simulink model "waypoint_generation_ptCloud_200630_waypoint_filtering_2"  (R2020a)
settings: Solver=ode4  StartTime=0.0  StopTime=200  FixedStep=0.01  RelTol=1e-3  EnableMultiTasking=on
InitFcn:
  | detector = load('ptOPDetector.mat');
  | OPdetector = detector.OPdetector;
undefined symbols (not defined in the file): g, Kd_p, Kd_q, Kd_r, Kd_vx, Kd_vy, Kd_vz, Kff_r, Kff_vx, Kff_vy, Kff_vz, Ki_p, Ki_q, Ki_r, Ki_vx, Ki_vy, Ki_vz, Kp_p, Kp_phi, Kp_psi, Kp_q, Kp_r, Kp_theta, Kp_vx, Kp_vy, Kp_vz, M, pointCloud_center, sigma_motor, w_h
libraries: visiontextngfix x4, sharedtransform x1, shared6dof x1, simulink_extras x1
(part 2 of 2)

== matlab function waypoint_generation_ptCloud_200630_waypoint_filtering_2/3D A* Algorithm/MATLAB Function11 ==
  settings: updateMethod=DISCRETE
  data: pos_grid input; waypoint_given input; point_cmd output; waypoint_gen input; auto_flag output; waypoint_set output
function [point_cmd,auto_flag,waypoint_set] = gen_waypoint(pos_grid,waypoint_given,waypoint_gen)

persistent flag autonomous_mode_flag waypoint_old waypoint_pre

if isempty(flag)
    flag = 1;
end
if isempty(autonomous_mode_flag)
    autonomous_mode_flag = 0;
end
if isempty(waypoint_old)
    waypoint_old = nan(20,3);
end
if isempty(waypoint_pre)
    waypoint_pre = nan(20,3);
    for aaa = 1:numel(waypoint_given)/3
        waypoint_pre(aaa,:)=waypoint_given(aaa,:);
    end
end
pos_grid = int32(pos_grid);
waypoint_pre_x = waypoint_pre(:,1);
waypoint_pre_y = waypoint_pre(:,2);
waypoint_pre_z = waypoint_pre(:,3);

point_cmd_temp = int32([waypoint_pre_x(flag) waypoint_pre_y(flag) waypoint_pre_z(flag)]);
waypoint_auto_set = nan(40,3);
waypoint_distance = nan(40,1);

if autonomous_mode_flag==0
    if abs(point_cmd_temp(1)-pos_grid(1)) <= 0 && abs(point_cmd_temp(2)-pos_grid(2)) <= 0 && abs(point_cmd_temp(3)-pos_grid(3)) <= 0
        flag = flag + 1;
        
        if flag == numel(rmmissing(waypoint_pre))/3 + 1
            flag = numel(rmmissing(waypoint_pre))/3;
            autonomous_mode_flag = 1;
        end
    end
    
    % waypoint_gen_filtered = rmmissing(waypoint_gen);
    % if ~isempty(waypoint_gen_filtered)
    %     if flag == numel(waypoint_pre)/3
    %         waypoint_x = waypoint_gen_filtered(1,1);
    %         waypoint_y = waypoint_gen_filtered(1,2);
    %         waypoint_z = waypoint_gen_filtered(1,3);
    %     end
    % end
elseif autonomous_mode_flag==1
    waypoint_auto_old = rmmissing(waypoint_old);
    waypoint_auto_new = rmmissing(waypoint_gen);
    if isempty(waypoint_auto_old)
        waypoint_auto_old = waypoint_auto_new;
    end
    
    if ~isempty(waypoint_auto_old) && ~isempty(waypoint_auto_new)
        for mmm = numel(waypoint_auto_new)/3:-1:1
            changed_flag=0;
            for nnn = 1:numel(waypoint_auto_old)/3
                if ((waypoint_auto_new(mmm,1)-waypoint_auto_old(nnn,1))^2+(waypoint_auto_new(mmm,2)-waypoint_auto_old(nnn,2))^2+(waypoint_auto_new(mmm,3)-waypoint_auto_old(nnn,3))^2)<900
                    waypoint_auto_old(nnn,:)=waypoint_auto_new(mmm,:);
                    changed_flag=1;
                end
            end
            if changed_flag == 1
                waypoint_auto_new(mmm,:)=nan(1,3);
            end
        end
%         waypoint_auto_set_temp = cat(1,unique(waypoint_auto_old,'stable','rows'),waypoint_auto_new);

%             waypoint_auto_set_temp = rmmissing(cat(1,waypoint_auto_new,unique(waypoint_auto_old,'stable','rows')));
            waypoint_auto_set_temp = rmmissing(cat(1,unique(waypoint_auto_old,'stable','rows'),waypoint_auto_new));

        
        for aaa = 1:numel(waypoint_auto_set_temp)/3
            waypoint_auto_set(aaa,:)=waypoint_auto_set_temp(aaa,:);
            waypoint_distance(aaa) = (((waypoint_auto_set(aaa,1)-pos_grid(1))^2+(waypoint_auto_set(aaa,2)-pos_grid(2))^2+(waypoint_auto_set(aaa,3)-pos_grid(3))^2));
        end
        [~,waypoint_index]=sort(waypoint_distance);
        
        for aaa = 1:length(waypoint_index)
            waypoint_auto_set(aaa,:)=waypoint_auto_set(waypoint_index(aaa),:);
        end
%         waypoint_auto_set(1:aaa,:)=waypoint_auto_set_temp(waypoint_index,:);
        
        point_cmd_temp = int32([waypoint_auto_set(1,1), waypoint_auto_set(1,2), waypoint_auto_set(1,3)]);
        
        if abs(point_cmd_temp(1)-pos_grid(1)) <= 0 && abs(point_cmd_temp(2)-pos_grid(2)) <= 0 && abs(point_cmd_temp(3)-pos_grid(3)) <= 0
            waypoint_auto_set = [waypoint_auto_set(2:end,:); nan(1,3)];            
        end
        
        waypoint_old = waypoint_auto_set(1:20,:);
        
        
    else
        if ~isnan(waypoint_old(1,1)) && ~isnan(waypoint_old(1,2)) && ~isnan(waypoint_old(1,3))
            point_cmd_temp = int32([waypoint_old(1,1), waypoint_old(1,2), waypoint_old(1,3)]);
%             waypoint_pre = waypoint_old;
%             autonomous_mode_flag = 0;
%             flag = 1;

            if abs(point_cmd_temp(1)-pos_grid(1)) <= 0 && abs(point_cmd_temp(2)-pos_grid(2)) <= 0 && abs(point_cmd_temp(3)-pos_grid(3)) <= 0
                waypoint_old = [waypoint_old(2:end,:); nan(1,3)];            
            end


        else
            point_cmd_temp = int32([pos_grid(1), pos_grid(2), pos_grid(3)]);
        end
    end
end


% point_cmd = int32([waypoint_pre_x(flag) waypoint_pre_y(flag) waypoint_pre_z(flag)]);
point_cmd = point_cmd_temp;


auto_flag = autonomous_mode_flag;
waypoint_set = waypoint_auto_set;


end

== matlab function waypoint_generation_ptCloud_200630_waypoint_filtering_2/3D A* Algorithm/MATLAB Function12 ==
  data: odom_input input; pos_grid output; pos_init input
function pos_grid = odom_grid(odom_input,pos_init)

odom = zeros(1,3);
odom(1,1) = odom_input(1);
odom(1,2) = odom_input(2);
odom(1,3) = odom_input(3);

start_point = [pos_init(1) pos_init(2) pos_init(3)];

% pos_x = int16(odom(1)/0.2+0.5);
% pos_y = int16(odom(2)/0.2+0.5);
% pos_z = int16(odom(3)/0.2+0.5);
pos_x = int16(odom(1)/0.2);
pos_y = int16(odom(2)/0.2);
pos_z = int16(odom(3)/0.2);

pos_grid = [pos_x+start_point(1) pos_y+start_point(2) pos_z+start_point(3)];

end

== matlab function waypoint_generation_ptCloud_200630_waypoint_filtering_2/3D A* Algorithm/MATLAB Function6 ==
  data: pos_init input; openpoint_front input; waypoint_gen output; openpoint_back input; openpoint_left input; openpoint_right input
function waypoint_gen = fcn(pos_init,openpoint_front,openpoint_back,openpoint_left,openpoint_right)
grid_size = 0.2;

openpoint_front_grid = int16(openpoint_front/grid_size);
openpoint_back_grid = int16(openpoint_back/grid_size);
openpoint_left_grid = int16(openpoint_left/grid_size);
openpoint_right_grid = int16(openpoint_right/grid_size);

waypoint_gen_front = nan(5,3);
waypoint_gen_back = nan(5,3);
waypoint_gen_left = nan(5,3);
waypoint_gen_right = nan(5,3);

for aaa = 1:5
    if ~isnan(openpoint_front(aaa,1))
        waypoint_gen_front(aaa,:) = [openpoint_front_grid(aaa,1)+int16(pos_init(1)), openpoint_front_grid(aaa,2)+int16(pos_init(2)), openpoint_front_grid(aaa,3)+int16(pos_init(3))];
    end
    if ~isnan(openpoint_back(aaa,1))
        waypoint_gen_back(aaa,:) = [openpoint_back_grid(aaa,1)+int16(pos_init(1)), openpoint_back_grid(aaa,2)+int16(pos_init(2)), openpoint_back_grid(aaa,3)+int16(pos_init(3))];
    end
    if ~isnan(openpoint_left(aaa,1))
        waypoint_gen_left(aaa,:) = [openpoint_left_grid(aaa,1)+int16(pos_init(1)), openpoint_left_grid(aaa,2)+int16(pos_init(2)), openpoint_left_grid(aaa,3)+int16(pos_init(3))];
    end
    if ~isnan(openpoint_right(aaa,1))
        waypoint_gen_right(aaa,:) = [openpoint_right_grid(aaa,1)+int16(pos_init(1)), openpoint_right_grid(aaa,2)+int16(pos_init(2)), openpoint_right_grid(aaa,3)+int16(pos_init(3))];
    end
end

waypoint_gen = [waypoint_gen_front;waypoint_gen_back;waypoint_gen_left;waypoint_gen_right];

== matlab function waypoint_generation_ptCloud_200630_waypoint_filtering_2/3D A* Algorithm/MATLAB Function9 ==
  data: bboxes_raw input; bboxes output; bboxes_size input
function bboxes = fcn(bboxes_raw,bboxes_size)
bboxes = zeros(5,4);
% bboxes_nonzeros = nonzeros(bboxes_raw);
% num_bboxes = min(numel(bboxes_nonzeros)/4,5);
num_bboxes = bboxes_size(1);

if num_bboxes>0
    for aaa = 1:num_bboxes
        bboxes(aaa,:) = [bboxes_raw(aaa+0*num_bboxes),bboxes_raw(aaa+1*num_bboxes),bboxes_raw(aaa+2*num_bboxes),bboxes_raw(aaa+3*num_bboxes)];
%         bboxes(aaa,:) = [bboxes_nonzeros(aaa+0*num_bboxes),bboxes_nonzeros(aaa+1*num_bboxes),bboxes_nonzeros(aaa+2*num_bboxes),bboxes_nonzeros(aaa+3*num_bboxes)];
    end
end
% bboxes(1:num_bboxes,:) = reshape(bboxes_nonzeros,num_bboxes,4);

== matlab function waypoint_generation_ptCloud_200630_waypoint_filtering_2/3D A* Algorithm/MATLAB Function10 ==
  data: bboxes_raw input; bboxes output; bboxes_size input
function bboxes = fcn(bboxes_raw,bboxes_size)
bboxes = zeros(5,4);
% bboxes_nonzeros = nonzeros(bboxes_raw);
% num_bboxes = min(numel(bboxes_nonzeros)/4,5);
num_bboxes = bboxes_size(1);

if num_bboxes>0
    for aaa = 1:num_bboxes
        bboxes(aaa,:) = [bboxes_raw(aaa+0*num_bboxes),bboxes_raw(aaa+1*num_bboxes),bboxes_raw(aaa+2*num_bboxes),bboxes_raw(aaa+3*num_bboxes)];
%         bboxes(aaa,:) = [bboxes_nonzeros(aaa+0*num_bboxes),bboxes_nonzeros(aaa+1*num_bboxes),bboxes_nonzeros(aaa+2*num_bboxes),bboxes_nonzeros(aaa+3*num_bboxes)];
    end
end
% bboxes(1:num_bboxes,:) = reshape(bboxes_nonzeros,num_bboxes,4);

== matlab function waypoint_generation_ptCloud_200630_waypoint_filtering_2/3D A* Algorithm/MATLAB Function13 ==
  data: bboxes_raw input; bboxes output; bboxes_size input
function bboxes = fcn(bboxes_raw,bboxes_size)
bboxes = zeros(5,4);
% bboxes_nonzeros = nonzeros(bboxes_raw);
% num_bboxes = min(numel(bboxes_nonzeros)/4,5);
num_bboxes = bboxes_size(1);

if num_bboxes>0
    for aaa = 1:num_bboxes
        bboxes(aaa,:) = [bboxes_raw(aaa+0*num_bboxes),bboxes_raw(aaa+1*num_bboxes),bboxes_raw(aaa+2*num_bboxes),bboxes_raw(aaa+3*num_bboxes)];
%         bboxes(aaa,:) = [bboxes_nonzeros(aaa+0*num_bboxes),bboxes_nonzeros(aaa+1*num_bboxes),bboxes_nonzeros(aaa+2*num_bboxes),bboxes_nonzeros(aaa+3*num_bboxes)];
    end
end
% bboxes(1:num_bboxes,:) = reshape(bboxes_nonzeros,num_bboxes,4);

== matlab function waypoint_generation_ptCloud_200630_waypoint_filtering_2/Generation_Angle_error/Attitude Generation (phi,theta,psi) ==
  data: DCM input; acc_cmd input; angle_error output; R_rp_x output
function [angle_error,R_rp_x]  = fcn(DCM,acc_cmd)
%#codegen

R_z           = DCM(3,:)'; 

% for i = 1:length(R_z)
%     if abs(R_z(i)) < 0.001
%         R_z(i) = 0;
%     end
% end

acc_unit      = R_z     / norm(R_z);
acc_cmd_unit  = acc_cmd / norm(acc_cmd);

angle_error = DCM * cross(acc_unit,acc_cmd_unit); %% e_R , consider phi, theta


% Calculate R_rp_x
angle = atan(norm(cross(acc_unit,acc_cmd_unit))/norm(dot(acc_unit,acc_cmd_unit))); % only phi,theta

e_R = angle_error;
R= DCM';

% e_R_cp matrix cross product
e_R_cp = zeros(3,3);
e_R_cp(1,2) = -e_R(3);
e_R_cp(1,3) =  e_R(2);
e_R_cp(2,1) =  e_R(3);
e_R_cp(2,3) = -e_R(1);
e_R_cp(3,1) = -e_R(2);
e_R_cp(3,2) =  e_R(1);

% Result
R_rp = R*(eye(3,3) + e_R_cp*sin(angle) + e_R_cp*e_R_cp*(1-cos(angle)));
R_rp_x = R_rp(:,1);
% acc_cmd_result = R_rp(:,3);

== matlab function waypoint_generation_ptCloud_200630_waypoint_filtering_2/3D A* Algorithm/MATLAB Function14 ==
  data: bboxes_raw input; bboxes output; bboxes_size input
function bboxes = fcn(bboxes_raw,bboxes_size)
bboxes = zeros(5,4);
% bboxes_nonzeros = nonzeros(bboxes_raw);
% num_bboxes = min(numel(bboxes_nonzeros)/4,5);
num_bboxes = bboxes_size(1);

if num_bboxes>0
    for aaa = 1:num_bboxes
        bboxes(aaa,:) = [bboxes_raw(aaa+0*num_bboxes),bboxes_raw(aaa+1*num_bboxes),bboxes_raw(aaa+2*num_bboxes),bboxes_raw(aaa+3*num_bboxes)];
%         bboxes(aaa,:) = [bboxes_nonzeros(aaa+0*num_bboxes),bboxes_nonzeros(aaa+1*num_bboxes),bboxes_nonzeros(aaa+2*num_bboxes),bboxes_nonzeros(aaa+3*num_bboxes)];
    end
end
% bboxes(1:num_bboxes,:) = reshape(bboxes_nonzeros,num_bboxes,4);

== matlab function waypoint_generation_ptCloud_200630_waypoint_filtering_2/3D A* Algorithm/MATLAB Function7 ==
  settings: updateMethod=DISCRETE
  data: pos_current input; optimal_path_x output size=[128 1]; point_cmd input; Obstacle input; pos_init input; optimal_path_y output size=[128 1]; optimal_path_z output size=[128 1]
function [optimal_path_x,optimal_path_y,optimal_path_z] = Astar_algorithm_function(pos_current,point_cmd,Obstacle,pos_init)

persistent optimal sample

if isempty(optimal)
    optimal = nan(128,3);
    sample = 99;
%     sample = 19;
end


sample = sample + 1;

if sample == 100
% if sample == 20
    sample = 1;
    
    mapsize = [150 100 30];
    
    Height = mapsize(1);        % x
    Width = mapsize(2);         % y
    Alt = mapsize(3);            % z
    
    Start = pos_current;
    Goal = point_cmd;
    look = 2;
    H_weight = 1.2;
    
    G_cost = zeros(2*look+1,2*look+1,2*look+1);
    for i = 1:2*look+1
        for j = 1:2*look+1
            for k = 1:2*look+1
                temp = [look+1 look+1 look+1]-[i j k];
                G_cost(i,j,k) = (min(sqrt(sum(abs(temp).^2,2))));
            end
        end
    end
    
    G_top2 = G_cost(:,:,1);
    G_top1 = G_cost(:,:,2);
    G_mid = G_cost(:,:,3);
    G_bottom1 = G_cost(:,:,4);
    G_bottom2 = G_cost(:,:,5);
    
    
    GScore = inf(Height,Width,Alt);
    GScore_temp = zeros(2*look+1,2*look+1,2*look+1);
    HScore = zeros(Height,Width,Alt);
    FScore = inf(Height,Width,Alt);
    ClosedMAT = zeros(Height,Width,Alt);
    CX = int32(Start(1));
    CY = int32(Start(2));
    CZ = int32(Start(3));
    ParentX = inf(Height,Width,Alt);
    ParentY = inf(Height,Width,Alt);
    ParentZ = inf(Height,Width,Alt);
    ParentX(CX,CY,CZ) = CX;
    ParentY(CX,CY,CZ) = CY;
    ParentZ(CX,CY,CZ) = CZ;
    
    %%%%%%%%%%%%%%%% Define Heuristic %%%%%%%%%%%%%%%%%%%%%%%
    for k=1:Alt
        for j=1:Width
            for i=1:Height
                
                temp = (int32(Goal) - int32([i j k])) ;
                Distance=(min(sqrt(sum(abs(temp).^2,2))));
                HScore(i,j,k)=Distance*H_weight;               % (1+sqrt(2))/sqrt(3)
                
            end
        end
    end
    
    FScore(Start(1),Start(2),Start(3)) = HScore(Start(1),Start(2),Start(3));
    GScore(Start(1),Start(2),Start(3)) = 0;
    ClosedMAT(Obstacle==1)=1;
    REACHGOAL = 0;
    
    while 1
        
        MinFScore = min(min(min(FScore)));         % Find Minimun FScore
        if isinf(MinFScore)
            disp('Fail');
            break
        end
        
        
        [minF_x,minF_y] = find(FScore==MinFScore);
        HScore_temp = inf(1,10);
        
        minHScore = 1;
        for i = 1:length(minF_x)
            Current_pose_temp = [minF_x(i) rem(minF_y(i),Width) fix(minF_y(i)/Width)+1];     % H가 가장 적은걸로 먼저 선택
            CX_temp=Current_pose_temp(1);
            CY_temp=Current_pose_temp(2);
            CZ_temp=Current_pose_temp(3);
            HScore_temp(i) = HScore(CX_temp,CY_temp,CZ_temp);
            minHScore = find(HScore_temp == min(HScore_temp));
        end
        
        
        Current_pose = int32([minF_x(minHScore(1)) rem(minF_y(minHScore(1)),Width) fix(minF_y(minHScore(1))/Width)+1]);     % H가 가장 적은걸로 먼저 선택
        CX=Current_pose(1);
        CY=Current_pose(2);
        CZ=Current_pose(3);
        
        
        
        GScore_temp(:,:,1) = GScore(CX,CY,CZ) + G_top2;
        GScore_temp(:,:,2) = GScore(CX,CY,CZ) + G_top1;
        GScore_temp(:,:,3) = GScore(CX,CY,CZ) + G_mid;
        GScore_temp(:,:,4) = GScore(CX,CY,CZ) + G_bottom1;
        GScore_temp(:,:,5) = GScore(CX,CY,CZ) + G_bottom2;
        
        
        
        
        %%%%%%%%%%%%% GScore update %%%%%%%%%%%%%
        
        GScore(CX-look:CX+look,CY-look:CY+look,CZ+2) = min(GScore_temp(:,:,1),GScore(CX-look:CX+look,CY-look:CY+look,CZ+2)) ;
        GScore(CX-look:CX+look,CY-look:CY+look,CZ+1) = min(GScore_temp(:,:,2),GScore(CX-look:CX+look,CY-look:CY+look,CZ+1));
        GScore(CX-look:CX+look,CY-look:CY+look,CZ) = min(GScore_temp(:,:,3), GScore(CX-look:CX+look,CY-look:CY+look,CZ));
        GScore(CX-look:CX+look,CY-look:CY+look,CZ-1) = min(GScore_temp(:,:,4),GScore(CX-look:CX+look,CY-look:CY+look,CZ-1));
        GScore(CX-look:CX+look,CY-look:CY+look,CZ-2) = min(GScore_temp(:,:,5),GScore(CX-look:CX+look,CY-look:CY+look,CZ-2));
        
        
        FScore = GScore + HScore;
        %     ClosedMAT(CX,CY,CZ) = 1;
        ClosedMAT(CX-(look-1):CX+(look-1),CY-(look-1):CY+(look-1),CZ-(look-1):CZ+(look-1)) = 1;
        FScore(ClosedMAT==1) = inf;
        %     Check_FScore = FScore(CX-look:CX+look,CY-look:CY+look,CZ-look:CZ+look);
        
        
        
        [G_row1,G_col1] = find( GScore(CX-look:CX+look,CY-look:CY+look,CZ+2) == GScore_temp(:,:,1) );
        [G_row2,G_col2] = find( GScore(CX-look:CX+look,CY-look:CY+look,CZ+1) == GScore_temp(:,:,2) );
        [G_row3,G_col3] = find( GScore(CX-look:CX+look,CY-look:CY+look,CZ) == GScore_temp(:,:,3) );
        [G_row4,G_col4] = find( GScore(CX-look:CX+look,CY-look:CY+look,CZ-1) == GScore_temp(:,:,4) );
        [G_row5,G_col5] = find( GScore(CX-look:CX+look,CY-look:CY+look,CZ-2) == GScore_temp(:,:,5) );
        
        
        G_row1 = int32(G_row1);
        G_row2 = int32(G_row2);
        G_row3 = int32(G_row3);
        G_row4 = int32(G_row4);
        G_row5 = int32(G_row5);
        
        G_col1 = int32(G_col1);
        G_col2 = int32(G_col2);
        G_col3 = int32(G_col3);
        G_col4 = int32(G_col4);
        G_col5 = int32(G_col5);
        
        G_row1 = G_row1+CX-(look+1);
        G_row2 = G_row2+CX-(look+1);
        G_row3 = G_row3+CX-(look+1);
        G_row4 = G_row4+CX-(look+1);
        G_row5 = G_row5+CX-(look+1);
        
        G_col1 = G_col1+CY-(look+1);
        G_col2 = G_col2+CY-(look+1);
        G_col3 = G_col3+CY-(look+1);
        G_col4 = G_col4+CY-(look+1);
        G_col5 = G_col5+CY-(look+1);
        
        
        for i = 1:length(G_row1)
            ParentX(G_row1(i),G_col1(i),CZ+2) = CX;
            ParentY(G_row1(i),G_col1(i),CZ+2) = CY;
            ParentZ(G_row1(i),G_col1(i),CZ+2) = CZ;
        end
        
        for i = 1:length(G_row2)
            ParentX(G_row2(i),G_col2(i),CZ+1) = CX;
            ParentY(G_row2(i),G_col2(i),CZ+1) = CY;
            ParentZ(G_row2(i),G_col2(i),CZ+1) = CZ;
        end
        
        for i = 1:length(G_row3)
            if G_row3(i)==CX && G_col3(i)==CY
                continue
            end
            ParentX(G_row3(i),G_col3(i),CZ) = CX;
            ParentY(G_row3(i),G_col3(i),CZ) = CY;
            ParentZ(G_row3(i),G_col3(i),CZ) = CZ;
        end
        
        for i = 1:length(G_row4)
            ParentX(G_row4(i),G_col4(i),CZ-1) = CX;
            ParentY(G_row4(i),G_col4(i),CZ-1) = CY;
            ParentZ(G_row4(i),G_col4(i),CZ-1) = CZ;
        end
        
        for i = 1:length(G_row5)
            ParentX(G_row5(i),G_col5(i),CZ-2) = CX;
            ParentY(G_row5(i),G_col5(i),CZ-2) = CY;
            ParentZ(G_row5(i),G_col5(i),CZ-2) = CZ;
        end
        
        
        
        
        if abs(Goal(1)-CX)<=(look-1) && abs(Goal(2)-CY)<=(look-1) && abs(Goal(3)-CZ)<=(look-1)
            REACHGOAL = 1;
            break
        end
        
    end
    
    
    % optimal = nan(128,3);
    if REACHGOAL
        optimal(1,:) = [Goal(1) Goal(2) Goal(3)];
        k=2;
        while 1
            CX_temp = int32(ParentX(CX,CY,CZ));
            CY_temp = int32(ParentY(CX,CY,CZ));
            CZ_temp = int32(ParentZ(CX,CY,CZ));
            
            CX = CX_temp;
            CY = CY_temp;
            CZ = CZ_temp;
            
            optimal(k,:) = [CX CY CZ];
            k = k+1;
            
            if CX==Start(1) && CY==Start(2) && CZ==Start(3)
                break
            end
        end
    end
    
end
start_point = [pos_init(1) pos_init(2) pos_init(3)];

% optimal_path_x = flip(single(((optimal(:,1)-start_point(1))-0.5) * 0.2 + 0.1));      % grid_size = 0.2
% optimal_path_y = flip(single(((optimal(:,2)-start_point(2))-0.5) * 0.2 + 0.1));
% optimal_path_z = flip(single(((optimal(:,3)-start_point(3))-0.5) * 0.2 + 0.1));
optimal_path_x = flip(single( (optimal(:,1)-start_point(1)) * 0.2 ));      % grid_size = 0.2
optimal_path_y = flip(single( (optimal(:,2)-start_point(2)) * 0.2 ));
optimal_path_z = flip(single( (optimal(:,3)-start_point(3)) * 0.2 ));


end

== matlab function waypoint_generation_ptCloud_200630_waypoint_filtering_2/3D A* Algorithm/MATLAB Function8 ==
  data: octomap_center input; Obstacle output; pos_init input
function Obstacle = gen_3d_array(octomap_center,pos_init)

mapsize = [150 100 30];

Obstacle = int8(zeros(mapsize(1),mapsize(2),mapsize(3)));
grid_size = 0.2;
start_point = [pos_init(1) pos_init(2) pos_init(3)];

% align1 = int16(octomap_center/(grid_size)+0.5);
align1 = int16(octomap_center/(grid_size));
align2 = unique(align1,'rows');
align3 = [align2(:,1)+start_point(1) align2(:,2)+start_point(2) align2(:,3)+start_point(3)];

for i = 1:numel(align3)/3
    
    index_temp = align3(i,:);
    
    index_check = index_temp<3;
    if sum(index_check)>=1
        index_temp(index_check) = 3;
    end
    
    if index_temp(1) > mapsize(1)-2
        index_temp(1) = mapsize(1)-2;
    end
    if index_temp(2) > mapsize(2)-2
        index_temp(2) = mapsize(2)-2;
    end
    if index_temp(3) > mapsize(3)-2
        index_temp(3) = mapsize(3)-2;
    end
    

    index_x = index_temp(1)-1:index_temp(1)+1;
    index_y = index_temp(2)-1:index_temp(2)+1;
    index_z = index_temp(3)-1:index_temp(3)+1;

    Obstacle(index_x,index_temp(2)+1,index_temp(3)+1) = 1;
    Obstacle(index_x,index_temp(2)+1,index_temp(3)) = 1;
    Obstacle(index_x,index_temp(2)+1,index_temp(3)-1) = 1;
    Obstacle(index_x,index_temp(2),index_temp(3)+1) = 1;
    Obstacle(index_x,index_temp(2),index_temp(3)) = 1;
    Obstacle(index_x,index_temp(2),index_temp(3)-1) = 1;
    Obstacle(index_x,index_temp(2)-1,index_temp(3)+1) = 1;
    Obstacle(index_x,index_temp(2)-1,index_temp(3)) = 1;
    Obstacle(index_x,index_temp(2)-1,index_temp(3)-1) = 1;
    
%     Obstacle(index_temp(1)+1,index_temp(2)+2,index_z) = 1;
%     Obstacle(index_temp(1)+1,index_temp(2)-2,index_z) = 1;
%     Obstacle(index_temp(1)+1,index_y,index_temp(3)+2) = 1;
%     Obstacle(index_temp(1)+1,index_y,index_temp(3)-2) = 1;
%     Obstacle(index_temp(1),index_temp(2)+2,index_z) = 1;
%     Obstacle(index_temp(1),index_temp(2)-2,index_z) = 1;
%     Obstacle(index_temp(1),index_y,index_temp(3)+2) = 1;
%     Obstacle(index_temp(1),index_y,index_temp(3)-2) = 1;
%     Obstacle(index_temp(1)-1,index_temp(2)+2,index_z) = 1;
%     Obstacle(index_temp(1)-1,index_temp(2)-2,index_z) = 1;
%     Obstacle(index_temp(1)-1,index_y,index_temp(3)+2) = 1;
%     Obstacle(index_temp(1)-1,index_y,index_temp(3)-2) = 1;
    
    
    
    
%     Obstacle(index_temp(1)+2,index_temp(2)+2,index_z) = 1;
%     Obstacle(index_temp(1)+2,index_temp(2)+1,index_z) = 1;
%     Obstacle(index_temp(1)+2,index_temp(2),index_z) = 1;
%     Obstacle(index_temp(1)+2,index_temp(2)-1,index_z) = 1;
%     Obstacle(index_temp(1)+2,index_temp(2)-2,index_z) = 1;
%     
%     Obstacle(index_temp(1)+1,index_temp(2)+2,index_z) = 1;
%     Obstacle(index_temp(1)+1,index_temp(2)+1,index_z) = 1;
%     Obstacle(index_temp(1)+1,index_temp(2),index_z) = 1;
%     Obstacle(index_temp(1)+1,index_temp(2)-1,index_z) = 1;
%     Obstacle(index_temp(1)+1,index_temp(2)-2,index_z) = 1;
%     
%     Obstacle(index_temp(1),index_temp(2)+2,index_z) = 1;
%     Obstacle(index_temp(1),index_temp(2)+1,index_z) = 1;
%     Obstacle(index_temp(1),index_temp(2),index_z) = 1;
%     Obstacle(index_temp(1),index_temp(2)-1,index_z) = 1;
%     Obstacle(index_temp(1),index_temp(2)-2,index_z) = 1;
%     
%     Obstacle(index_temp(1)-1,index_temp(2)+2,index_z) = 1;
%     Obstacle(index_temp(1)-1,index_temp(2)+1,index_z) = 1;
%     Obstacle(index_temp(1)-1,index_temp(2),index_z) = 1;
%     Obstacle(index_temp(1)-1,index_temp(2)-1,index_z) = 1;
%     Obstacle(index_temp(1)-1,index_temp(2)-2,index_z) = 1;
%     
%     Obstacle(index_temp(1)-2,index_temp(2)+2,index_z) = 1;
%     Obstacle(index_temp(1)-2,index_temp(2)+1,index_z) = 1;
%     Obstacle(index_temp(1)-2,index_temp(2),index_z) = 1;
%     Obstacle(index_temp(1)-2,index_temp(2)-1,index_z) = 1;
%     Obstacle(index_temp(1)-2,index_temp(2)-2,index_z) = 1;
    
end

Obstacle(1:3,:,:)=1;
Obstacle(mapsize(1)-2:mapsize(1),:,:) = 1;
Obstacle(:,1:3,:) = 1;
Obstacle(:,mapsize(2)-2:mapsize(2),:) = 1;
Obstacle(:,:,1:3) = 1;
Obstacle(:,:,mapsize(3)-10:mapsize(3)) = 1;

end

== matlab function waypoint_generation_ptCloud_200630_waypoint_filtering_2/Path Guidance/MATLAB Function ==
  data: X_vel_cmd output; Y_vel_cmd output; odom input; Z_vel_cmd output; optimal_path_x input size=[128 1]; optimal_path_y input size=[128 1]; optimal_path_z input size=[128 1]; yaw_cmd output
function [X_vel_cmd,Y_vel_cmd,Z_vel_cmd,yaw_cmd] = fcn(odom,optimal_path_x,optimal_path_y,optimal_path_z)

P_gain = 0.5;

path_length = length(optimal_path_x);
K = inf(path_length,1);
optimal_path_norm = inf(path_length,3);

% optimal_path_x_temp = optimal_path_x.Data';
% optimal_path_y_temp = optimal_path_y.Data';

optimal_path_norm(:,1) = single(optimal_path_x - odom(1));
optimal_path_norm(:,2) = single(optimal_path_y - odom(2));
optimal_path_norm(:,3) = single(optimal_path_z - odom(3));

% optimal_path = [optimal_path_x' optimal_path_y'];
% optimal_path_norm = optimal_path - [odom(1) odom(2)];

for i=1:path_length
    K(i) = norm(optimal_path_norm(i,:));
end

[~,m] = min(K);



% Z_cmd = optimal_path_z(m);
if m >= 128
    m = 127;
end
% Z_cmd = optimal_path_z(m+1) + APF_vector(3);         % prediction
% X_cmd = optimal_path_x(m+1) + APF_vector(1);
% Y_cmd = optimal_path_y(m+1) + APF_vector(2);
Z_cmd = optimal_path_z(m+1);       
X_cmd = optimal_path_x(m+1);
Y_cmd = optimal_path_y(m+1);

error_z = (Z_cmd - odom(3));
error_x = (X_cmd - odom(1));
error_y = (Y_cmd - odom(2));

Z_vel_cmd = double(error_z*P_gain);
X_vel_cmd = double(error_x*P_gain);
Y_vel_cmd = double(error_y*P_gain);
% yaw_cmd = atan2(Y_cmd-odom(2),X_cmd-odom(1));        % 고쳐야함 
% yaw_cmd = atan2(optimal_path_y(m+1)-odom(2),optimal_path_x(m+1)-odom(1)); 
if m <= 125
    yaw_vector1 = [optimal_path_x(m+1)-odom(1) optimal_path_y(m+1)-odom(2)] / norm([optimal_path_x(m+1)-odom(1) optimal_path_y(m+1)-odom(2)]);
    yaw_vector2 = [optimal_path_x(m+2)-odom(1) optimal_path_y(m+2)-odom(2)] / norm([optimal_path_x(m+2)-odom(1) optimal_path_y(m+2)-odom(2)]);
    yaw_vector3 = [optimal_path_x(m+3)-odom(1) optimal_path_y(m+3)-odom(2)] / norm([optimal_path_x(m+3)-odom(1) optimal_path_y(m+3)-odom(2)]);
    yaw_vector = yaw_vector1 + yaw_vector2 + yaw_vector3;
    yaw_cmd = double( atan2(yaw_vector(2),yaw_vector(1)) );
%     yaw_cmd = double( ( atan2(optimal_path_y(m+1)-odom(2),optimal_path_x(m+1)-odom(1)) + atan2(optimal_path_y(m+2)-odom(2),optimal_path_x(m+2)-odom(1)) + atan2(optimal_path_y(m+3)-odom(2),optimal_path_x(m+3)-odom(1)) ) / 3 );
else
    yaw_cmd = 0;
end

end

== matlab function waypoint_generation_ptCloud_200630_waypoint_filtering_2/Motor_Dynamics/Motor Dynamics/Motor Rotation Speed Generation ==
  data: w_dot_cmd input; w_state input; w_motor output; T_require output; Moment output; w_motor_square output; a_cmd input; DCM input
function [w_motor,T_require,Moment,w_motor_square] = fcn(w_dot_cmd,w_state,a_cmd,DCM)

w_motor        = zeros(4,1);
% ============= Quadrotor Spec  ==========================================%
kafa_f = 6.41*10^-6;                    % thrust coefficient
kafa_tau = 1.69*10^-2;                  % moment coefficient

L = 0.22/2;                               % length ( motor to motor) [m]
M = 0.5 ; %mass    [Kg]

I_T = [3.2*10^-3,3.2*10^-3,5.5*10^-3];  % total moment
I_P = [0,0,1.5*10^-5];                  % propeller reaction moment
I_B = I_T - 4*I_P;                      % frame inertia moment
Inertia = diag(I_B);
% 
% T_require = M * norm(a_cmd);
T_hover = [0,0,1]; %Thrust
R_z = DCM(:,3);
g = 9.8; %gravity [m/s^2]
T_require = M*(abs(a_cmd) / dot(T_hover,R_z));


Moment = Inertia*w_dot_cmd + cross(w_state,Inertia*w_state);

A = [1       ,  1         ,   1         ,   1;
    0        ,  L         ,   0         ,  -L;
    -L       ,  0         ,   L         ,   0;
    kafa_tau , -kafa_tau  ,   kafa_tau  ,  -kafa_tau];

w_motor_square = A^-1 * [T_require;Moment]/kafa_f;

for i = 1:length(w_motor_square)
    w_motor(i) = sqrt(abs(w_motor_square(i)));
end

== matlab function waypoint_generation_ptCloud_200630_waypoint_filtering_2/Quadrotor Dynamics/중력항 고려 ==
  data: Mg input; DCM_e2b input; Fe output
function Fe = fcn(Mg,DCM_e2b)

Fe=DCM_e2b*Mg;

== matlab function waypoint_generation_ptCloud_200630_waypoint_filtering_2/Generation_Angle_error/Attitude Generation(psi^*) ==
  data: R_rp_x input; acc_cmd input; Bearing_angle input; psi_angle_error output
function psi_angle_error   = fcn(R_rp_x,acc_cmd,Bearing_angle)
%#codegen

acc_cmd_unit  = acc_cmd / norm(acc_cmd); % define hat(k)_B_des
sigma = Bearing_angle;

j_sigma_des = [-sin(sigma),cos(sigma),0]; % hat(i)_sigma_des

i_B_des =  cross(j_sigma_des,acc_cmd_unit);
R_sp_x  =  i_B_des;
% 
% temp  = cross(R_rp_x,R_sp_x);
% temp2 = dot(R_rp_x,R_sp_x);

psi_angle_error = atan(cross(R_rp_x,R_sp_x)*acc_cmd_unit/dot(R_rp_x,R_sp_x))*acc_cmd_unit(3)^2;

% psi_angle_error = atan(norm(cross(R_rp_x,R_sp_x))/dot(R_rp_x,R_sp_x));

== matlab function waypoint_generation_ptCloud_200630_waypoint_filtering_2/Generation_Angle_error/Attitude Generation(phi,theta,psi^*) ==
  data: angle_error input; psi_angle_error input; angle_error_result output
function angle_error_result  = fcn(angle_error,psi_angle_error)
%#codegen

angle_error_result = [angle_error(1);angle_error(2);psi_angle_error];

% if norm(temp) ~= 0
%     angle_error_result  = temp / norm(temp);
% else
%     angle_error_result  = temp;
% end

== matlab function waypoint_generation_ptCloud_200630_waypoint_filtering_2/MATLAB Function ==
  settings: updateMethod=DISCRETE
  data: current_pos input; pointCloud_current output size=[500000 3]; pointCloud_center input
function pointCloud_current = fcn(current_pos, pointCloud_center)

persistent pointCloud_old block_hz
if isempty(block_hz)
    block_hz = 5;
end
pointCloud_center = double(pointCloud_center);

size_max = 500000;
filtering_distance = 8; %m

pointCloud_new = nan(size_max,3);
pointCloud_current = nan(size_max,3);

% if block_hz ==5
%     block_hz = 0;
    for aaa = 1:numel(pointCloud_center)/3
        if sqrt((pointCloud_center(aaa,1)-current_pos(1))^2+(pointCloud_center(aaa,2)-current_pos(2))^2+(pointCloud_center(aaa,3)-current_pos(3))^2)<filtering_distance
            %         pointCloud_new = cat(1,pointCloud_new,pointCloud_center(aaa,:));
            pointCloud_new(aaa,:) = pointCloud_center(aaa,:);
        end
    end
    
    if isempty(pointCloud_old)
        pointCloud_old = nan(size_max,3);
    end
    
    pointCloud_temp=cat(1,rmmissing(pointCloud_old),rmmissing(pointCloud_new));
    pointCloud_unique = unique(pointCloud_temp,'rows');
    % pointCloud_current=cat(1,cat(1,rmmissing(pointCloud_old),rmmissing(pointCloud_new)),nan(100000-(numel(rmmissing(pointCloud_old))/3+numel(rmmissing(pointCloud_new))/3),3));
    % pointCloud_current=[rmmissing(pointCloud_temp);nan(200000-numel(rmmissing(pointCloud_temp))/3,3)];
    for aaa = 1:numel(pointCloud_unique)/3
        if (~isnan(pointCloud_unique(aaa,1)))&&(~isnan(pointCloud_unique(aaa,2)))&&(~isnan(pointCloud_unique(aaa,3)))
            pointCloud_current(aaa,:)=pointCloud_unique(aaa,:);
        end
    end
    
    
% end

pointCloud_old = pointCloud_current;
% block_hz = block_hz +1;

== matlab function waypoint_generation_ptCloud_200630_waypoint_filtering_2/Quadrotor Dynamics/Translation body -> Earth ==
  data: Ab input; DCM input; Ae output
function Ae = fcn(Ab,DCM)
%#codegen

ax_b = Ab(1);
ay_b = Ab(2);
az_b = Ab(3);

a_b = [ax_b;ay_b;az_b];
Ae = DCM'*a_b;

== matlab function waypoint_generation_ptCloud_200630_waypoint_filtering_2/Position_Controller/Velocity Controller/Acceleration Saturation ==
  data: a_cmd input; a_cmd_sat output; a_norm output
function [a_cmd_sat,a_norm] = fcn(a_cmd)
%#codegen

tilt_max = 35*pi/180; % [rad  ] , tolerant tilt , user define
thr_max  = 11;        % [m/s^2] , tolerant acceleration , user define (90% maximum, 50% hovering)
% thr_max  = 9.8/50 * 90; 

thrust_sp_xy_len = norm([a_cmd(1) a_cmd(2)]);
thrust_xy_max    = abs(a_cmd(3)) * tan(tilt_max);

if thrust_sp_xy_len >= thrust_xy_max
    k =  thrust_xy_max/thrust_sp_xy_len;
    a_cmd_sat = [a_cmd(1)*k ; a_cmd(2)*k ; a_cmd(3)];
else
    a_cmd_sat = a_cmd;
end


if a_cmd_sat(3)/abs(a_cmd_sat(3)) >= 0 
    if abs(a_cmd_sat(3)) >= thr_max

        k  = a_cmd_sat(3) / abs(a_cmd_sat(3));
        a_cmd_sat = [0 ; 0 ; k*thr_max];
    else
        thrust_sp_xy_len_sat = sqrt(a_cmd_sat(1)^2 + a_cmd_sat(2)^2);
        thrust_xy_max_sat    = sqrt(-a_cmd_sat(3)^2 + thr_max^2); 

        if thrust_sp_xy_len_sat >= thrust_xy_max_sat
            k = thrust_xy_max_sat / thrust_sp_xy_len_sat;
            a_cmd_sat = [a_cmd_sat(1)*k ; a_cmd_sat(2)*k ; a_cmd_sat(3)];
        end
    end
else
    a_cmd_sat = [a_cmd_sat(1) ; a_cmd_sat(2) ; 0.00001];
end

a_norm = norm(a_cmd_sat);

== matlab function waypoint_generation_ptCloud_200630_waypoint_filtering_2/Path Guidance/MATLAB Function1 ==
  data: w input; yaw output; x input; y input; z input
function yaw = quat2yaw(w,x,y,z)

euler_angle = quat2eul([w x y z],'ZYX');
yaw = euler_angle(1);
end
